simulink model "Psim"  (R2015a)
settings: Solver=ode3  StartTime=0.0  StopTime=inf  FixedStep=0.0001  RelTol=1e-3
libraries: xpcquanserlib x4, slrtlib x2
settings Model: SimulationMode=external  CovSFcnEnable=off  Creator=Venkatraman  LastModifiedBy=trupal
settings SolverCC: EnableConcurrentExecution=on
settings OptimizationCC: BlockReduction=off  OptimizeBlockIOStorage=off  BufferReuse=off  GlobalBufferReuse=off  ExpressionFolding=off  LocalBlockOutputs=off
settings DebuggingCC: SolverPrmCheckMsg=warning
settings HardwareCC: ProdIntDivRoundTo=Zero  ProdEndianess=LittleEndian  ProdLongLongMode=on  ProdHWDeviceType=Generic->32-bit x86 compatible  TargetLongLongMode=on  TargetIntDivRoundTo=Zero  TargetEndianess=LittleEndian  TargetHWDeviceType=MATLAB Host
settings RTWCC: SystemTargetFile=slrt.tlc  TemplateMakefile=slrt_default_tmf  Description=Simulink Real-Time  RTWVerbose=off  RTWCompilerOptimization=on
settings SimulinkRealTimeCC: GeneratePreprocessorConditionals=Disable all

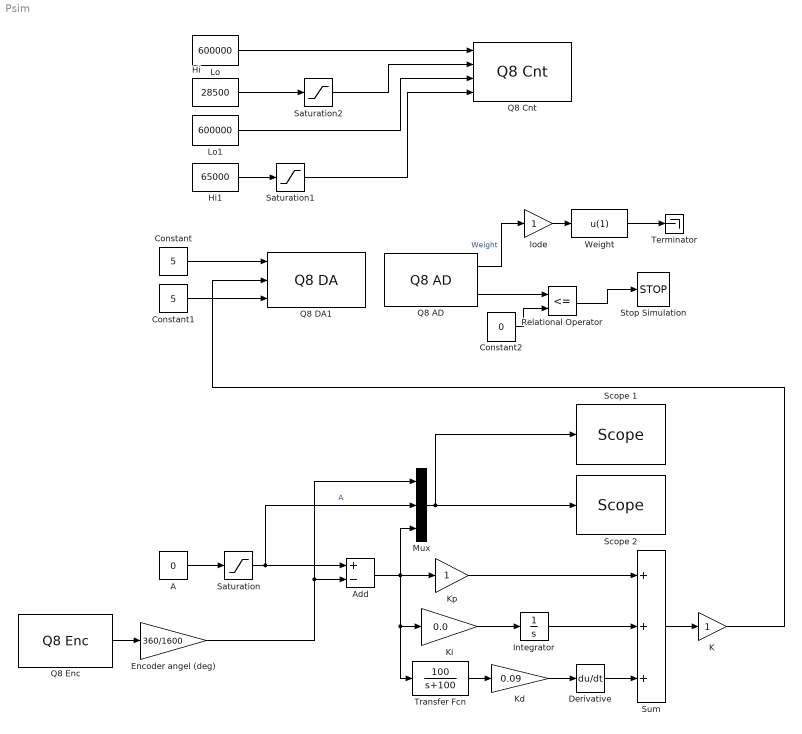
== system Psim ==
  A : Constant  Value=0
  Add : Sum  Inputs=+-
  Constant : Constant  Value=5
  Constant1 : Constant  Value=5
  Constant2 : Constant  Value=0
  Derivative : Derivative
  Encoder angel (deg) : Gain  Gain=360/1600
  Hi : Constant  Value=28500
  Hi1 : Constant  Value=65000
  Integrator : Integrator
  K : Gain
  Kd : Gain  Gain=0.09
  Ki : Gain  Gain=0.0
  Kp : Gain
  Lo : Constant  Value=600000
  Lo1 : Constant  Value=600000
  Mux : Mux  Inputs=3
  Q8 AD : xpcquanserlib/A//D/Q8 AD  channel=[1,5]  sampleTime=-1  slot=-1
  Q8 Cnt : xpcquanserlib/Counter/Q8 Cnt  channel=[1,2]  mode=[1]  showArm=[0]  reset=[1]  initLoCount=[0]  initHiCount=[0]  sampleTime=-1  slot=-1
  Q8 DA1 : xpcquanserlib/D//A/Q8 DA  channel=[5,3,2]  range=[-5]  simul=off  reset=[1]  initValue=[0]  sampleTime=-1  slot=-1
  Q8 Enc : xpcquanserlib/Incremental Encoder/Q8 Enc  channel=[1]  initialCount=[0]  prescale=[1]  quadrature=[4]  mode=[0]  synchronousIndex=[0]  indexPolarity=[0]  preserveCounts=[0]  sampleTime=-1  slot=-1
  Relational Operator : RelationalOperator  Operator=<=  OutDataTypeStr=boolean
  Saturation : Saturate  UpperLimit=0  LowerLimit=-270-48
  Saturation1 : Saturate  UpperLimit=65000  LowerLimit=33000
  Saturation2 : Saturate  UpperLimit=30000  LowerLimit=20000
  Scope 1 : slrtlib/Displays and Logging/Scope   scopeno=1  scopetype=Host  autostart=on  viewmode=Graphical redraw  formatstr='%15.6f'  grid=on  ylimits=[0,0]  nosamples=1000  noprepostsamples=0  interleave=1  triggermode=Signal triggering  triggersignal=2  trigsignalfromport=off  triggerlevel=1  triggerslope=Either  triggerscope=1  triggersample=0  filename=data.dat  mode=Lazy  writesize=512  autorestart=off  dynamicfilemode=off  maxwritefilesize=512*1024^2
  Scope 2 : slrtlib/Displays and Logging/Scope   scopeno=2  scopetype=Target  autostart=on  viewmode=Graphical redraw  formatstr='%15.6f'  grid=on  ylimits=[0,180]  nosamples=250  noprepostsamples=0  interleave=1  triggermode=FreeRun  triggersignal=2  trigsignalfromport=off  triggerlevel=1  triggerslope=Either  triggerscope=1  triggersample=0  filename=data.dat  mode=Lazy  writesize=512  autorestart=off  dynamicfilemode=off  maxwritefilesize=512*1024^2
  Stop Simulation : Stop
  Sum : Sum  Inputs=+++
  Terminator : Terminator
  Transfer Fcn : TransferFcn  Numerator=[100]  Denominator=[1 100]
  Weight : Fcn  Expr=u(1)
  lode : Gain
  wires:
  Saturation/1 -> Add/1, Mux/2  "A"
  Q8 Enc/1 -> Encoder angel (deg)/1
  Encoder angel (deg)/1 -> Add/2, Mux/1
  Add/1 -> Mux/3, Transfer Fcn/1, Ki/1, Kp/1
  Ki/1 -> Integrator/1
  Transfer Fcn/1 -> Kd/1
  Kd/1 -> Derivative/1
  Derivative/1 -> Sum/3
  Integrator/1 -> Sum/2
  Kp/1 -> Sum/1
  Sum/1 -> K/1
  Mux/1 -> Scope 2/1, Scope 1/1
  Lo/1 -> Q8 Cnt/1
  Hi/1 -> Saturation2/1
  Constant/1 -> Q8 DA1/1
  Relational Operator/1 -> Stop Simulation/1
  Constant2/1 -> Relational Operator/2
  K/1 -> Q8 DA1/2
  Constant1/1 -> Q8 DA1/3
  A/1 -> Saturation/1
  Q8 AD/2 -> Relational Operator/1
  Q8 AD/1 -> lode/1  "Weight"
  Lo1/1 -> Q8 Cnt/3
  Hi1/1 -> Saturation1/1
  Saturation1/1 -> Q8 Cnt/4
  Saturation2/1 -> Q8 Cnt/2
  lode/1 -> Weight/1
  Weight/1 -> Terminator/1
